simulink model "gm_LogicProcessor"  (R2016a)
settings: Solver=FixedStepDiscrete  SolverMode=SingleTasking  StartTime=0.0  StopTime=1000  RelTol=1e-3
libraries: hdlsllib x2
settings Model: Creator=sande  LastModifiedBy=sande
settings SolverCC: AutoInsertRateTranBlk=on
settings DataIOCC: LimitDataPoints=on  SaveFormat=Array  SaveOutput=off  SaveTime=off
settings OptimizationCC: BlockReduction=off  ConditionallyExecuteInputs=off  DefaultParameterBehavior=Inlined  UseDivisionForNetSlopeComputation=UseDivisionForReciprocalsOfIntegersOnly  UseFloatMulNetSlope=on  InlineInvariantSignals=on  EnhancedBackFolding=on  EfficientFloat2IntCast=on  OptimizeModelRefInitCode=on  LifeSpan=1
settings DebuggingCC: AlgebraicLoopMsg=error  SolverPrmCheckMsg=warning  InheritedTsInSrcMsg=none  SingleTaskRateTransMsg=error  AllowSymbolicDim=off  StrictBusMsg=ErrorOnBusTreatedAsVector  NonBusSignalsTreatedAsBus=error
settings HardwareCC: ProdBitPerPointer=32  ProdLargestAtomicFloat=None  ProdIntDivRoundTo=Undefined  ProdEndianess=Unspecified  ProdWordSize=32  ProdHWDeviceType=ASIC/FPGA->ASIC/FPGA  ProdEqTarget=off
settings ModelReferenceCC: PropagateSignalLabelsOutOfModel=off
settings RTWCC: SystemTargetFile=ert.tlc  TemplateMakefile=ert_default_tmf  GenerateReport=on  IncludeHyperlinkInReport=on  LaunchReport=on  GenerateTraceInfo=on  GenerateTraceReport=on  GenerateTraceReportSl=on  GenerateTraceReportSf=on  GenerateTraceReportEml=on  GenerateCodeMetricsReport=on
settings CodeAppCC: IgnoreCustomStorageClasses=off
settings ERTTargetCC: GenerateSampleERTMain=on  CombineSignalStateStructs=on  SuppressErrorStatus=on  InlinedParameterPlacement=NonHierarchical  ERTCustomFileTemplate=example_file_process.tlc  ConvertIfToSwitch=off  SuppressUnreachableDefaultCases=off
settings ConfigComp: CovModelRefEnable=Off  CovSFcnEnable=off

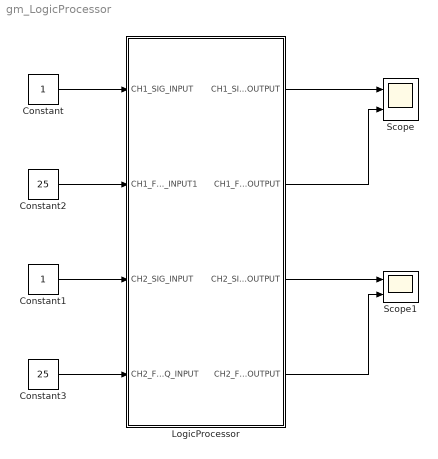
== system gm_LogicProcessor ==
  Constant : Constant  OutDataTypeStr=boolean  SampleTime=1
  Constant1 : Constant  OutDataTypeStr=boolean  SampleTime=1
  Constant2 : Constant  Value=25  OutDataTypeStr=uint32  SampleTime=1
  Constant3 : Constant  Value=25  OutDataTypeStr=uint32  SampleTime=1
  LogicProcessor : Subsystem
  Scope : Scope  NumInputPorts=2
  Scope1 : Scope  NumInputPorts=2
  wires:
  Constant3/1 -> LogicProcessor/4(CH2_FREQ_INPUT)
  Constant2/1 -> LogicProcessor/2(CH1_FREQ_INPUT1)
  Constant1/1 -> LogicProcessor/3(CH2_SIG_INPUT)
  LogicProcessor/4(CH2_FREQ_OUTPUT) -> Scope1/2
  LogicProcessor/3(CH2_SIG_OUTPUT) -> Scope1/1
  LogicProcessor/2(CH1_FREQ_OUTPUT) -> Scope/2
  LogicProcessor/1(CH1_SIG_OUTPUT) -> Scope/1
  Constant/1 -> LogicProcessor/1(CH1_SIG_INPUT)

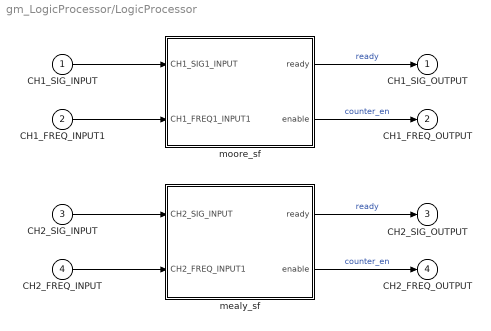
== system gm_LogicProcessor/LogicProcessor ==
  CH1_SIG_INPUT : Inport
  CH1_FREQ_INPUT1 : Inport  Port=2
  CH2_SIG_INPUT : Inport  Port=3
  CH2_FREQ_INPUT : Inport  Port=4
  mealy_sf : Subsystem
  moore_sf : Subsystem
  CH1_SIG_OUTPUT : Outport
  CH1_FREQ_OUTPUT : Outport  Port=2
  CH2_SIG_OUTPUT : Outport  Port=3
  CH2_FREQ_OUTPUT : Outport  Port=4
  wires:
  CH2_FREQ_INPUT/1 -> mealy_sf/2(CH2_FREQ_INPUT1)
  CH1_FREQ_INPUT1/1 -> moore_sf/2(CH1_FREQ1_INPUT1)
  CH1_SIG_INPUT/1 -> moore_sf/1(CH1_SIG1_INPUT)
  mealy_sf/2(enable) -> CH2_FREQ_OUTPUT/1  "counter_en"
  mealy_sf/1(ready) -> CH2_SIG_OUTPUT/1  "ready"
  moore_sf/1(ready) -> CH1_SIG_OUTPUT/1  "ready"
  CH2_SIG_INPUT/1 -> mealy_sf/1(CH2_SIG_INPUT)
  moore_sf/2(enable) -> CH1_FREQ_OUTPUT/1  "counter_en"

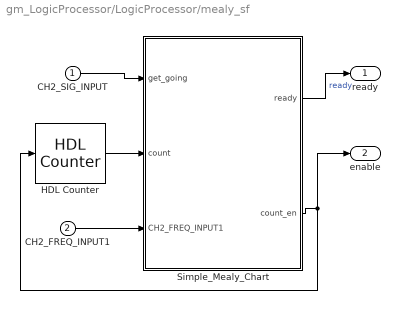
== system gm_LogicProcessor/LogicProcessor/mealy_sf ==
  CH2_SIG_INPUT : Inport
  CH2_FREQ_INPUT1 : Inport  Port=2
  HDL Counter : hdlsllib/HDL Operations/HDL Counter  CountType=Count limited  CountInit=0  CountStep=1  CountMax=25  CountFromType=Initial value  CountFrom=0  CountResetPort=off  CountLoadPort=off  CountEnbPort=on  CountDirPort=off  CountDataType=Unsigned  CountWordLen=8  CountFracLen=0  CountSampTime=1
  Simple_Mealy_Chart : Stateflow chart  TreatAsAtomicUnit=on
  ready : Outport
  enable : Outport  Port=2
  wires:
  CH2_FREQ_INPUT1/1 -> Simple_Mealy_Chart/3(CH2_FREQ_INPUT1)
  HDL Counter/1 -> Simple_Mealy_Chart/2(count)
  Simple_Mealy_Chart/2(count_en) -> HDL Counter/1, enable/1
  Simple_Mealy_Chart/1(ready) -> ready/1  "ready"
  CH2_SIG_INPUT/1 -> Simple_Mealy_Chart/1(get_going)

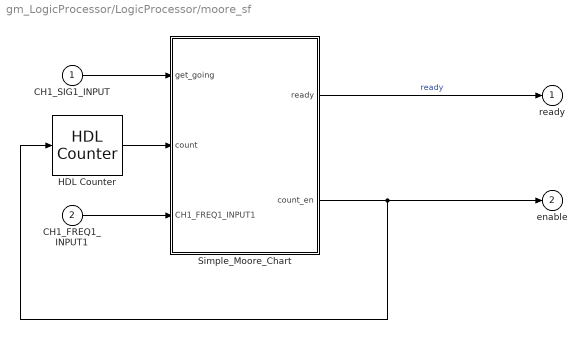
== system gm_LogicProcessor/LogicProcessor/moore_sf ==
  CH1_SIG1_INPUT : Inport
  CH1_FREQ1_INPUT1 : Inport  Port=2
  HDL Counter : hdlsllib/HDL Operations/HDL Counter  CountType=Count limited  CountInit=0  CountStep=1  CountMax=50  CountFromType=Initial value  CountFrom=0  CountResetPort=off  CountLoadPort=off  CountEnbPort=on  CountDirPort=off  CountDataType=Unsigned  CountWordLen=8  CountFracLen=0  CountSampTime=1
  Simple_Moore_Chart : Stateflow chart  TreatAsAtomicUnit=on
  ready : Outport
  enable : Outport  Port=2
  wires:
  CH1_FREQ1_INPUT1/1 -> Simple_Moore_Chart/3(CH1_FREQ1_INPUT1)
  CH1_SIG1_INPUT/1 -> Simple_Moore_Chart/1(get_going)
  Simple_Moore_Chart/1(ready) -> ready/1  "ready"
  HDL Counter/1 -> Simple_Moore_Chart/2(count)
  Simple_Moore_Chart/2(count_en) -> HDL Counter/1, enable/1

== stateflow chart gm_LogicProcessor/LogicProcessor/moore_sf/Simple_Moore_Chart ==
  settings: stateMachineType=MOORE_MACHINE  initializeOutput=1
  state IDLE
    ready = true;
    count_en = false;
  state COUNTING
    ready = false;
    count_en = true;
  (default) -> IDLE
  COUNTING -> IDLE : [(count) == CH1_FREQ1_INPUT1]
  IDLE -> COUNTING : [get_going == true]
  data: get_going input boolean; count input =0; ready output boolean =true; count_en output boolean; max_count constant fixdt(0,5,0) =25; CH1_FREQ1_INPUT1 input

== stateflow chart gm_LogicProcessor/LogicProcessor/mealy_sf/Simple_Mealy_Chart ==
  settings: stateMachineType=MEALY_MACHINE  executeAtInitialization=1
  state IDLE
  state COUNTING
  (default) -> IDLE
  COUNTING -> IDLE : [count == max_count]...
      | {ready = true;...
      | count_en = false;}
  IDLE -> COUNTING : [get_going == true]...
      | {ready = false;...
      |  count_en = true;}
  data: get_going input boolean; count input uint8 =0; ready output boolean =true; count_en output boolean; max_count constant uint8 =25; CH2_FREQ_INPUT1 input
